simulink model "1_Diode_rectifier"  (R2014a)
settings: Solver=ode23tb  StartTime=0.0  StopTime=2  RelTol=1e-6
libraries: powerlib x15, powerlib_meascontrol x1
settings Model: Creator=CHANDRA BABU  LastModifiedBy=Divya M
settings SolverCC: ZeroCrossControl=DisableAll
settings DataIOCC: SignalLoggingSaveFormat=ModelDataLogs
settings OptimizationCC: ExpressionDepthLimit=2147483647
settings DebuggingCC: UnderspecifiedInitializationDetection=Classic  FcnCallInpInsideContextMsg=UseLocalSettings  StateNameClashWarn=warning
settings GRTTargetCC: CombineOutputUpdateFcns=off  GRTInterface=on

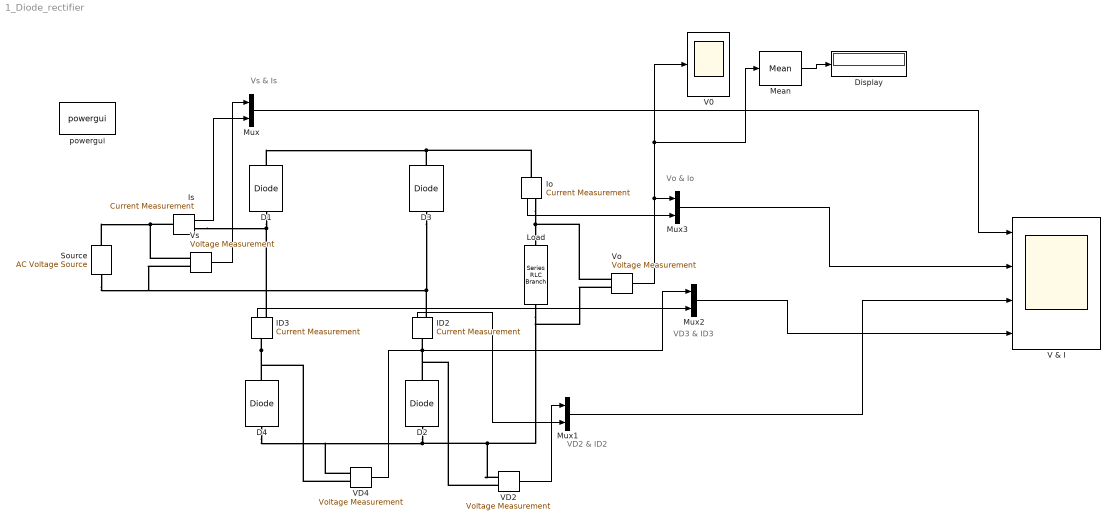
== system 1_Diode_rectifier ==
  note: Vo & Io
  note: VD3 & ID3
  note: VD2 & ID2
  note: Vs & Is
  " Source" : powerlib/Electrical Sources/AC Voltage Source  Amplitude=5  Phase=0  Frequency=50  SampleTime=0  Measurements=None
  D{1..4} (4 alike) : powerlib/Power Electronics/Diode  Ron=0.001  Lon=0  Vf=0  IC=0  UseSnubber=off  Rs=500  Cs=250e-9  Measurements=off
  Display : Display
  ID2 : powerlib/Measurements/Current Measurement  PhasorSimulation=off  OutputType=Complex  PSBequivalent=0
  ID3 : powerlib/Measurements/Current Measurement  PhasorSimulation=off  OutputType=Complex  PSBequivalent=0
  Io : powerlib/Measurements/Current Measurement  PhasorSimulation=off  OutputType=Complex  PSBequivalent=0
  Is : powerlib/Measurements/Current Measurement  PhasorSimulation=off  OutputType=Complex  PSBequivalent=0
  Load : powerlib/Elements/Series RLC Branch  LConnTagsString=__new0  RConnTagsString=__new0  BranchType=R  Resistance=2.5  Inductance=1e-3  SetiL0=off  InitialCurrent=0  Capacitance=1e-6  Setx0=off  InitialVoltage=0  Measurements=None
  Mean : powerlib_meascontrol/Measurements/Mean  Freq=60  Vinit=0  Ts=0
  Mux{,1..3} (4 alike) : Mux  Inputs=2
  V & I : Scope  NumInputPorts=4
      settings: YMin=-5~0~-5~-5  YMax=5~5~2~2
  V0 : Scope
      settings: SaveName=Outputvoltage
  VD2 : powerlib/Measurements/Voltage Measurement  PhasorSimulation=off  OutputType=Complex  PSBequivalent=0
  VD4 : powerlib/Measurements/Voltage Measurement  PhasorSimulation=off  OutputType=Complex  PSBequivalent=0
  Vo : powerlib/Measurements/Voltage Measurement  PhasorSimulation=off  OutputType=Complex  PSBequivalent=0
  Vs : powerlib/Measurements/Voltage Measurement  PhasorSimulation=off  OutputType=Complex  PSBequivalent=0
  powergui : powerlib/powergui  Priority=1  SimulationMode=Continuous  SolverType=Tustin  SampleTime=50e-6  frequency=60  SPID=off  DisableSnubberDevices=off  DisableRonSwitches=off  DisableVfSwitches=off  SwTol=0  Interpol=off  DisplayEquations=off  Ts=0  methode=off  frequencyindice=0  Pbase=100e6  ErrMax=1e-4  Iterations=50  UnitsV=kV  UnitsW=MW  FunctionMessages=off  echomessages=off  HookPort=off  EnableUseOfTLC=off  x0status=blocks  RestoreLinks=warning  ResistiveCurrentMeasurement=off  Frange=[0:2:500]  Ylog=off  Xlog=on  ShowGrid=off  save=off  variable=ZData  structure=Outputvoltage  ZoomFFT=on  StartTime=0.0  cycles=1  DisplayStyle=1  fundamental=50  FreqAxis=on  MaxFrequency=1000  frequencyindicesteady=1  RmsSteady=1  display=off
  wires:
  Vo/1 -> Mean/1, V0/1, Mux3/1
  Is/1 -> Mux/2
  VD2/1 -> Mux1/1
  ID3/1 -> Mux2/2
  Io/1 -> Mux3/2
  VD4/1 -> Mux2/1
  Vs/1 -> Mux/1
  ID2/1 -> Mux1/2
  Mux/1 -> V & I/1
  Mux3/1 -> V & I/2
  Mux1/1 -> V & I/3
  Mux2/1 -> V & I/4
  Mean/1 -> Display/1
  connections:
  D1/LConn1 -- Is/RConn1 -- ID3/RConn1
  ID3/LConn1 -- D4/RConn1 -- VD4/LConn2
  ID2/LConn1 -- D2/RConn1 -- VD2/LConn2
  Vs/LConn1 -- " Source"/RConn1 -- Is/LConn1
  D3/LConn1 -- ID2/RConn1 -- " Source"/LConn1 -- Vs/LConn2
  Vo/LConn1 -- Io/RConn1 -- Load/LConn1
  VD2/LConn1 -- Vo/LConn2 -- Load/RConn1 -- VD4/LConn1 -- D4/LConn1 -- D2/LConn1
  D1/RConn1 -- Io/LConn1 -- D3/RConn1
